simulink model "theta_control_hardware"  (R2025b)
settings: Solver=ode4  StartTime=0.0  StopTime=20000  FixedStep=0.001  RelTol=1e-3  EnableMultiTasking=on
settings Model: Creator=MarkMad  LastModifiedBy=MarkMad
settings SolverCC: AlgebraicLoopSolver=TrustRegion
settings DataIOCC: LimitDataPoints=on  ReturnWorkspaceOutputs=off
settings OptimizationCC: LifeSpan=inf
settings DebuggingCC: UnconnectedInputMsg=warning  UnconnectedOutputMsg=warning  UnconnectedLineMsg=warning  AllowSymbolicDim=off  SFUnexpectedBacktrackingDiag=warning  SFNoUnconditionalDefaultTransitionDiag=warning  SFExecutionAtInitializationDiag=none  ArithmeticOperatorsInVariantConditions=warning
settings ModelReferenceCC: EnableRefExpFcnMdlSchedulingChecks=on  PropagateSignalLabelsOutOfModel=off
settings SFSimCC: SimUseLocalCustomCode=off  CustomCodeUndefinedFunction=UseInterfaceOnly
settings RTWCC: RTWUseLocalCustomCode=off  GPUComputeCapability=3.5
settings CodeAppCC: StateflowObjectComments=on
settings GRTTargetCC: TargetLangStandard=C89/C90 (ANSI)
settings ConfigComp: CovMetricSettings=dw  CovSaveCumulativeToWorkspaceVar=on  CovSaveSingleToWorkspaceVar=on  CovExternalEMLEnable=off

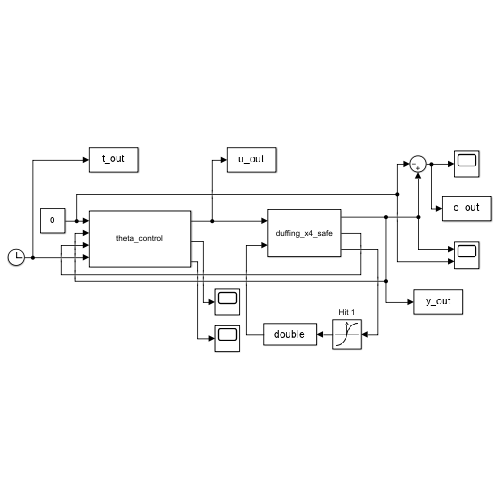
[thumbnail: Simulink's stored preview of the top-level diagram]
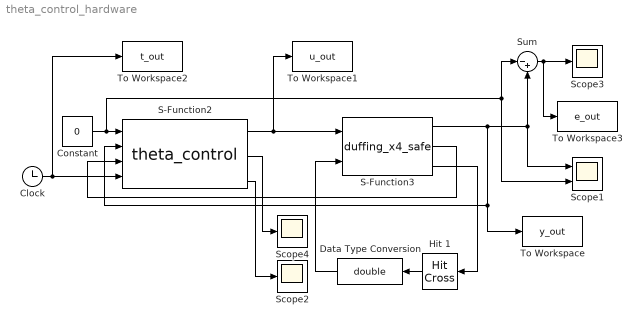
== system theta_control_hardware ==
  Clock : Clock
  Constant : Constant  Value=0
  Data Type Conversion : DataTypeConversion  OutDataTypeStr=double  SaturateOnIntegerOverflow=off  RndMeth=Floor
  Hit 1 : HitCross  HitCrossingOffset=2.0*pi  HitCrossingDirection=rising
  S-Function2 : S-Function  FunctionName=theta_control  Parameters=0.5, 0.15, 0.1  SFunctionDeploymentMode=off  EnableBusSupport=off
  S-Function3 : S-Function  FunctionName=duffing_x4_safe  Parameters="-0.2 -0.6   0.25 0.3  1.0"  SFunctionDeploymentMode=off  EnableBusSupport=off
  Scope1 : Scope  NumInputPorts=2
      settings: ActiveDisplayYMinimum=-0.34109  ActiveDisplayYMaximum=0.32048
  Scope2 : Scope
      settings: ActiveDisplayYMinimum=-0.0036260067605754279  ActiveDisplayYMaximum=0.003621384941892603  DataLoggingSaveFormat=Array
  Scope3 : Scope
      settings: ActiveDisplayYMinimum=-0.34109  ActiveDisplayYMaximum=0.32048
  Scope4 : Scope
      settings: ActiveDisplayYMinimum=-319.47887  ActiveDisplayYMaximum=708.38687
  Sum : Sum  Inputs=|-+
  To Workspace : ToWorkspace  VariableName=y_out  SampleTime=-1
  To Workspace1 : ToWorkspace  VariableName=u_out  SampleTime=-1
  To Workspace2 : ToWorkspace  VariableName=t_out  SampleTime=-1
  To Workspace3 : ToWorkspace  VariableName=e_out  SampleTime=-1
  wires:
  S-Function3/2 -> S-Function2/3
  Sum/1 -> Scope3/1, To Workspace3/1
  Clock/1 -> S-Function2/4, To Workspace2/1
  Constant/1 -> Scope1/2, Sum/1, S-Function2/1
  S-Function2/2 -> Scope4/1
  S-Function2/3 -> Scope2/1
  S-Function3/3 -> Hit 1/1
  Hit 1/1 -> Data Type Conversion/1
  Data Type Conversion/1 -> S-Function3/2
  S-Function3/1 -> Scope1/1, Sum/2, To Workspace/1, S-Function2/2
  S-Function2/1 -> S-Function3/1, To Workspace1/1
